simulink model "openloop_DE_B"  (R2017a)
settings: Solver=FixedStepDiscrete  StartTime=0.0  StopTime=Tf  FixedStep=Ts  RelTol=1e-3  EnableMultiTasking=on
values from neighbouring files (symbols this model uses):
  Ts = t(2)-t(1)    [check_filter.m]    (also in closedloop_driver.m = 0.1; openloop_driver.m = 0.1; wheel_parameters.m = 0.05)
libraries: simulink x2
settings Model: Creator=throne  LastModifiedBy=localmgr
settings DataIOCC: LimitDataPoints=on  SaveFormat=Array
settings OptimizationCC: ExpressionDepthLimit=2147483647  InitFltsAndDblsToZero=on  LifeSpan=inf
settings DebuggingCC: UnderspecifiedInitializationDetection=Classic  MergeDetectMultiDrivingBlocksExec=none  SolverPrmCheckMsg=warning  StateNameClashWarn=warning  SFUnexpectedBacktrackingDiag=warning  SFNoUnconditionalDefaultTransitionDiag=warning  SFExecutionAtInitializationDiag=none
settings HardwareCC: ProdBitPerPointer=32  ProdBitPerSizeT=32  ProdBitPerPtrDiffT=32  ProdLargestAtomicFloat=None  ProdIntDivRoundTo=Undefined  ProdEndianess=Unspecified  ProdWordSize=32  ProdHWDeviceType=32-bit Generic
settings ModelReferenceCC: PropagateSignalLabelsOutOfModel=off
settings GRTTargetCC: TargetLangStandard=C89/C90 (ANSI)  GeneratePreprocessorConditionals=Disable all  CombineOutputUpdateFcns=off  GRTInterface=on
settings ConfigComp: CovMetricSettings=dw  CovHtmlReporting=on  CovSaveCumulativeToWorkspaceVar=on  CovSaveSingleToWorkspaceVar=on  CovExternalEMLEnable=off

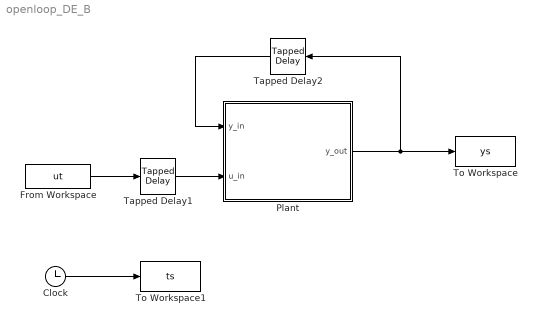
== system openloop_DE_B ==
  " Plant" : MATLAB Function  TreatAsAtomicUnit=on
  Clock : Clock
  From Workspace : FromWorkspace  VariableName=ut  SampleTime=0
  Tapped Delay1 : simulink/Discrete/Tapped Delay  vinit=0  samptime=Ts  NumDelays=1  DelayOrder=Newest  includeCurrent=off
  Tapped Delay2 : simulink/Discrete/Tapped Delay  vinit=0.0  samptime=-1  NumDelays=1  DelayOrder=Newest  includeCurrent=off
  To Workspace : ToWorkspace  VariableName=ys  SampleTime=-1
  To Workspace1 : ToWorkspace  VariableName=ts  SampleTime=Ts
  wires:
  Clock/1 -> To Workspace1/1
  Tapped Delay2/1 -> " Plant"/1(y_in)
  Tapped Delay1/1 -> " Plant"/2(u_in)
  From Workspace/1 -> Tapped Delay1/1
  " Plant"/1(y_out) -> To Workspace/1, Tapped Delay2/1

== matlab function openloop_DE_B/ Plant ==
  data: y_in input size=[1 1]; u_in input size=[1 2]; y_out output
function y_out  = fcn(y_in, u_in)
% This block supports the Embedded MATLAB subset.
% See the help menu for details. 
  y_out = 0.8*y_in(1)+1 - 0.2 * u_in(1);
